simulink model "qcar_sensor_validation"  (R2024b)
settings: Solver=ode1  StartTime=0.0  StopTime=inf  FixedStep=Controller_Sample_Time  RelTol=1e-3  EnableMultiTasking=on
undefined symbols (not defined in the file): AAAF5050, angles_qcar2, cal_pos, Controller_Sample_Time, CSI_Sample_Time, gcbh, GyroKF_P0, GyroKF_Q, GyroKF_R, GyroKF_X0, height, HIL, ImageDisplay_Sample_Time, Initialization_Time, JPEG, K12, left, LiDAR_Sample_Time, MC, path_x4, path_y4, Point, qc_get_step_size, qcar2_lidar_to_body_rotation, qcar2_lidar_to_map_rotation, qcar2_virtual_to_physical_lidar_rotation, QCarEKF_L, QCarEKF_P0, QCarEKF_Q, QCarEKF_R_combined, QCarEKF_R_heading, QcarKF_X0, range_qcar2, RealSense_Sample_Time, steering_Kd, steering_Kp, top, video_display_show, width
libraries: quarc_library x45, simulink_extras x6, simulink x3, mspfiltlib x1
(part 3 of 3)

== matlab function qcar_sensor_validation/obstacleDetection/obstacleDetection Markham March 22/Draw Lines Module ==
  data: img_in input; img_out output; pts input; color input
function img_out = drawLines(img_in, pts, color)

% Draw lines connecting the points using the provided color

% Inputs:
% u         : Input RGB Image (size = m by n)
% pts       : p x-y pairs of points (px) where markers are to be drawn
% color     : 1x3 matrix of RGB color values for each marker

% Outputs:
% y         : Output RGB Image with the markers drawn in (size = m by n)

%% Initialization
if size(img_in, 3) == 3
    img_out = img_in;
elseif size(img_in, 3) == 1
    img_out = cat(3, img_in, img_in, img_in);
end

[p, ~] = size(pts); % determine the number of points

%% Draw the lines
    for i = 1:p-1
        % determine the max(rows_difference, col_difference) between two
        % points
        itr = max(abs(pts(i,1) - pts(i+1,1)), abs(pts(i,2) - pts(i+1,2)));
        
        % generate linear spaces of row and col values between the pts
        row_vec = round(linspace(pts(i,1), pts(i+1,1), itr));
        col_vec = round(linspace(pts(i,2), pts(i+1,2), itr));
        
        % iterate through the values and shade them right

        for j = 1:itr
            img_out(row_vec(j), col_vec(j),1) = color(1);
            img_out(row_vec(j), col_vec(j),2) = color(2);
            img_out(row_vec(j), col_vec(j),3) = color(3);
        end
    end
end

== matlab function qcar_sensor_validation/obstacleDetection/obstacleDetection Markham March 22/Steering based image subselector ==
  data: pts output; depth input; distance output; steering input; minDistance input; maxDistance input; width input; height input; vertCenter input; maxSteering input; reduction input; maxSteeringWidth input
function [pts, distance] = estimateDepthInRegion(depth, steering, minDistance, maxDistance, width, height, vertCenter, maxSteering, reduction, maxSteeringWidth)
% Input: 640 x 360
[ROW, COL] = size(depth);
mark = COL/2 - (steering*(COL/2 - width/2)/maxSteering);
applied_width = max(width - abs(steering/maxSteeringWidth)*reduction*width, 60);
left_w = max(mark+1-(applied_width/2), 0); % pick the left end, but never let it get negative
right_w = min(left_w + applied_width, COL); % pick the right end, but never past the image width
upper_h = max(ROW*vertCenter-height/2+1, 0); % pick the upper end, but never let it get negative
lower_h = min(ROW*vertCenter+height/2, ROW); % pick the lower end, but never let it go past the image height
depth(:,1:40) = maxDistance; %this is to remove artifacts in the camera's left section
region = double(depth(upper_h:lower_h, left_w:right_w)); 
pts = [upper_h, left_w; upper_h, right_w; lower_h, right_w; lower_h, left_w; upper_h, left_w];
u_flat = reshape(region, 1, []);

temp = maxDistance*ones(1, length(u_flat));

for i = 1:length(u_flat)
    if (u_flat(i) >= minDistance) && (u_flat(i) <= maxDistance)
        temp(i) = u_flat(i);
    end
end

% u_flat(u_flat < minDistance) = [];
% u_flat(u_flat > maxDistance) = [];
% distance = mean(mean(u_flat));
distance = min(temp(:));
